simulink model "acrobot_zerodynamics_simulink_control"  (R2023a)
settings: Solver=ode45  StartTime=0.0  StopTime=10.0  MaxStep=1e-4  RelTol=1e-4
values from neighbouring files (symbols this model uses):
  k3 = 75    [acrobot_parameters.m]
  k4 = 50    [acrobot_parameters.m]
settings Model: Creator=MSI-  LastModifiedBy=MSI-

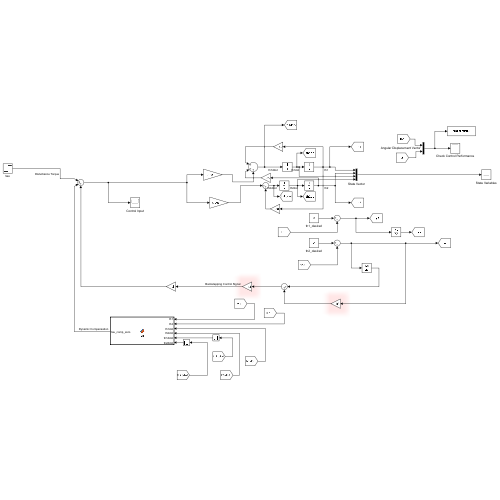
[thumbnail: Simulink's stored preview of the top-level diagram]
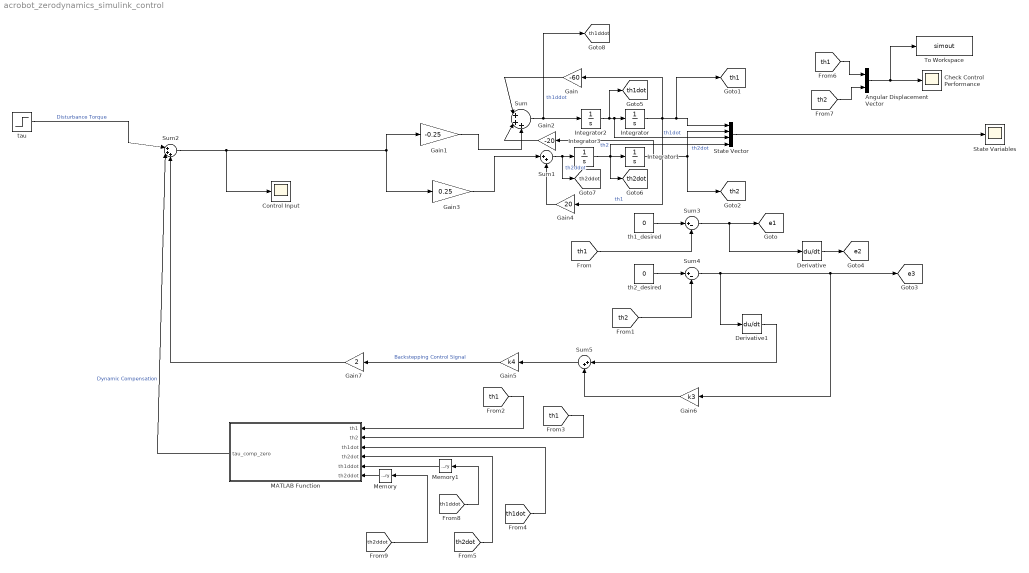
== system acrobot_zerodynamics_simulink_control ==
  Angular Displacement Vector : Mux  Inputs=2
  Check Control Performance : Scope
  Control Input : Scope
  Derivative : Derivative
  Derivative1 : Derivative
  Gain : Gain  Gain=-60
  Gain1 : Gain  Gain=-0.25
  Gain2 : Gain  Gain=-20
  Gain3 : Gain  Gain=0.25
  Gain4 : Gain  Gain=20
  Gain5 : Gain  Gain=k4
  Gain6 : Gain  Gain=k3
  Gain7 : Gain  Gain=2
  Integrator{,1..3} (4 alike) : Integrator
  MATLAB Function : MATLAB Function  TreatAsAtomicUnit=on
  Memory : Memory
  Memory1 : Memory
  State Variables : Scope
  State Vector : Mux
  Sum : Sum  Inputs=|+++
  Sum1 : Sum  Inputs=|++
  Sum2 : Sum  Inputs=|+++
  Sum3 : Sum  Inputs=|+-
  Sum4 : Sum  Inputs=|+-
  Sum5 : Sum  Inputs=|++
  To Workspace : ToWorkspace  VariableName=simout  SaveFormat=Timeseries  SampleTime=-1
  tau : Step  SampleTime=0
  th1_desired : Constant  Value=0
  th2_desired : Constant  Value=0
  tag scope: e1=global, e2=global, e3=global, th1=global, th1ddot=global, th1dot=global, th2=global, th2ddot=global, th2dot=global
  wires:
  State Vector/1 -> State Variables/1
  Integrator/1 -> Gain4/1, Gain/1, [th1], State Vector/1  "th1"
  Integrator1/1 -> Gain2/1, [th2], State Vector/2  "th2"
  Sum/1 -> [th1ddot], Integrator2/1  "th1ddot"
  Integrator2/1 -> [th1dot], State Vector/3, Integrator/1  "th1dot"
  Integrator3/1 -> [th2dot], State Vector/4, Integrator1/1  "th2dot"
  Gain/1 -> Sum/1
  Gain1/1 -> Sum/3
  Gain2/1 -> Sum/2
  Sum1/1 -> [th2ddot], Integrator3/1  "th2ddot"
  Gain4/1 -> Sum1/2
  Gain3/1 -> Sum1/1
  tau/1 -> Sum2/1  "Disturbance Torque"
  Sum2/1 -> Control Input/1, Gain1/1, Gain3/1
  th1_desired/1 -> Sum3/1
  th2_desired/1 -> Sum4/1
  Sum3/1 -> Derivative/1, [e1]
  [th1] -> Sum3/2
  [th2] -> Sum4/2
  Sum4/1 -> Derivative1/1, Gain6/1, [e3]
  Derivative/1 -> [e2]
  Derivative1/1 -> Sum5/1
  Gain6/1 -> Sum5/2
  Sum5/1 -> Gain5/1
  [th1] -> MATLAB Function/1(th1)
  [th1] -> MATLAB Function/2(th2)
  [th1dot] -> MATLAB Function/3(th1dot)
  [th2dot] -> MATLAB Function/4(th2dot)
  Gain5/1 -> Gain7/1  "Backstepping Control Signal"
  Angular Displacement Vector/1 -> To Workspace/1, Check Control Performance/1
  [th1] -> Angular Displacement Vector/1
  [th2] -> Angular Displacement Vector/2
  MATLAB Function/1(tau_comp_zero) -> Sum2/2  "Dynamic Compensation"
  [th2ddot] -> Memory/1
  [th1ddot] -> Memory1/1
  Gain7/1 -> Sum2/3
  Memory/1 -> MATLAB Function/6(th2ddot)
  Memory1/1 -> MATLAB Function/5(th1ddot)

== matlab function acrobot_zerodynamics_simulink_control/MATLAB Function ==
  data: th1 input; tau_comp_zero output; th2 input; th1dot input; th2dot input; th1ddot input; th2ddot input
function tau_comp_zero = fcn(th1,th2,th1dot,th2dot,th1ddot,th2ddot)
%tau_comp=((cos(th2) + 2)*(80*sin(th1) - sin(th1 + th2) + 4*th1dot*th2dot*sin(th2)*(2*th1dot + th2dot)))/(4*(cos(th2)^2 - 2)) - ((- 4*th2dot*sin(th2)*th1dot^2 + 80*sin(th1 + th2))*(2*cos(th2) + 3))/(4*(cos(th2)^2 - 2));
A=[0,0,1,0;0,0,0,1;-60,-20,0,0;20,0,0,0];
B=[0;0;-0.25;0.25];
xdot=[th1dot;th2dot;th1ddot;th2ddot];
x=[th1;th2;th1dot;th2dot];
tau_comp_zero=-pinv(B)*(xdot-A*x);
end
